simulink model "produce_sensor_fault_noise"  (Simulink 7.7)
settings: Solver=ode45  StartTime=0.0  StopTime=10.0  RelTol=1e-3
values from neighbouring files (symbols this model uses):
  Tsamp = 0.001    [LSDP_controllers_nntraining_data_igva.m]    (also in initialize_LSDP_controllers_igva.m)
libraries: simulink x2
settings Model: Creator=mk  LastModifiedBy=mk

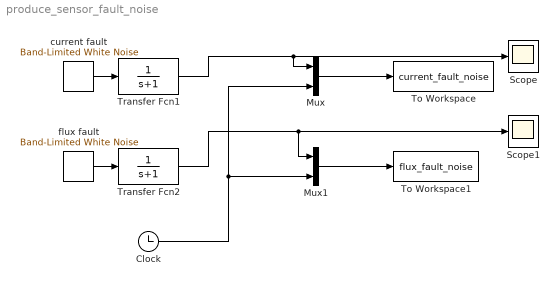
== system produce_sensor_fault_noise ==
  Clock : Clock
      settings: Decimation=10
  Mux : Mux  Inputs=2
  Mux1 : Mux  Inputs=2
  Scope : Scope
  Scope1 : Scope
  To Workspace : ToWorkspace  VariableName=current_fault_noise  SampleTime=-1  SaveFormat=Array
  To Workspace1 : ToWorkspace  VariableName=flux_fault_noise  SampleTime=-1  SaveFormat=Array
  Transfer Fcn1 : TransferFcn  Denominator=[1 1]
  Transfer Fcn2 : TransferFcn  Denominator=[1 1]
  current fault : simulink/Sources/Band-Limited White Noise  SystemSampleTime=-1  Cov=1  Ts=Tsamp  seed=[23341]
  flux fault : simulink/Sources/Band-Limited White Noise  SystemSampleTime=-1  Cov=0.00015  Ts=Tsamp  seed=[23341]
  wires:
  current fault/1 -> Transfer Fcn1/1
  flux fault/1 -> Transfer Fcn2/1
  Transfer Fcn1/1 -> Scope/1, Mux/1
  Transfer Fcn2/1 -> Scope1/1, Mux1/1
  Mux1/1 -> To Workspace1/1
  Mux/1 -> To Workspace/1
  Clock/1 -> Mux1/2, Mux/2
